simulink model "pilote_hydraulique_Stateflow_0"  (R2020a)
settings: Solver=ode23t  StartTime=0.0  StopTime=1500  RelTol=1e-3  EnableMultiTasking=on
undefined symbols (not defined in the file): sigbuilder_block, X, Y, Z
libraries: sm_lib x295, fl_lib x24, nesl_utility x13, sh_lib x5, simulink x1
(part 1 of 5)
settings Model: Creator=Ivan  LastModifiedBy=ivanl
settings DataIOCC: LimitDataPoints=on  SaveFormat=Array  ReturnWorkspaceOutputs=off
settings OptimizationCC: LifeSpan=inf
settings DebuggingCC: UnderspecifiedInitializationDetection=Classic  MergeDetectMultiDrivingBlocksExec=none  SolverPrmCheckMsg=warning  AllowSymbolicDim=off  StateNameClashWarn=warning  SFUnexpectedBacktrackingDiag=warning  SFNoUnconditionalDefaultTransitionDiag=warning  SFExecutionAtInitializationDiag=none  ArithmeticOperatorsInVariantConditions=warning
settings HardwareCC: ProdBitPerPointer=32  ProdBitPerSizeT=32  ProdBitPerPtrDiffT=32  ProdLargestAtomicFloat=None  ProdIntDivRoundTo=Undefined  ProdEndianess=Unspecified  ProdWordSize=32  ProdHWDeviceType=32-bit Generic
settings ModelReferenceCC: PropagateSignalLabelsOutOfModel=off
settings SFSimCC: SimUseLocalCustomCode=off  CustomCodeUndefinedFunction=UseInterfaceOnly
settings RTWCC: RTWUseLocalCustomCode=off
settings CodeAppCC: StateflowObjectComments=on
settings GRTTargetCC: TargetLangStandard=C89/C90 (ANSI)
settings ConfigComp: CovMetricSettings=dw  CovHtmlReporting=on  CovSaveCumulativeToWorkspaceVar=on  CovSaveSingleToWorkspaceVar=on  CovExternalEMLEnable=off
settings SimscapeCC: SimscapeNormalizeSystem=off  SimscapeLogType=all  SimscapeLogLimitData=off
settings ConfigurationSet: Description=SimMechanics 2G
settings ExplorerConfigSet: InternalSimMechanicsExplorerSettings="<ExplorerConfiguration><canonicalview>default</canonicalview><AnimationSetting><BasePlaybackSpeed>1.0</BasePlaybackSpeed><PlaybackSpeedFactor>16.0</PlaybackSpeedFactor></AnimationSetting><TilePanel><TileInfo><Tiles Columns=\"2\" Count=\"4\" Rows=\"2\"><Column Left=\"2\" Weight=\"0.5\"/><Column Left=\"554\" Weight=\"0.5\"/><Column Left=\"1106\"/><Row Top=\"2\" Weight=\"0.4992\"/><Row Top=\"320\" Weight=\"0.5008\"/><Row Top=\"639\"/><Tile Height=\"1\" Width=\"1\" X=\"0\" Y=\"0\"/><Tile Height=\"1\" Width=\"1\" X=\"0\" Y=\"1\"/><Tile Height=\"1\" Width=\"1\" X=\"1\" Y=\"0\"/><Tile Height=\"1\" Width=\"1\" X=\"1\" Y=\"1\"/></Tiles></TileInfo><SceneInfo><SceneViewer><BGColor><R>0.60000002384185791</R><G>0.60000002384185791</G><B>0.60000002384185791</B></BGColor><Camera><Position><X>-1.4545420789578025</X><Y>-0.47703526853152423</Y><Z>1.053292472596125</Z></Position><Center><X>-1.0755331343287176</X><Y>0.65681441625729753</Y><Z>0.33046154790126991</Z></Center><Up><X>0.31799715127972389</X><Y>0.43179203595848165</Y><Z>0.84405772874893448</Z></Up><Left>-0.52137946486473086</Left><Right>0.52137946486473086</Right><Bottom>-0.12744375988841058</Bottom><Top>0.12744375988841058</Top></Camera></SceneViewer><SceneViewer><BGColor><R>0.60000002384185791</R><G>0.60000002384185791</G><B>0.60000002384185791</B></BGColor><Camera><Position><X>-1.097124655307177</X><Y>0.60879350298107193</Y><Z>1.6773847746848054</Z></Position><Center><X>-1.097124655307177</X><Y>0.60879350298107193</Y><Z>0.3230140209197998</Z></Center><Up><X>0</X><Y>1</Y><Z>-0</Z></Up><Left>-0.52137946486473086</Left><Right>0.52137946486473086</Right><Bottom>-0.19162502065300943</Bottom><Top>0.19162502065300943</Top></Camera></SceneViewer><SceneViewer><BGColor><R>0.60000002384185791</R><G>0.60000002384185791</G><B>0.60000002384185791</B></BGColor><Camera><Position><X>-1.839713975613805</X><Y>1.4497817237667032</Y><Z>1.0667372871108483</Z></Position><Center><X>-1.0007040048852538</X><Y>0.55541256489420043</Y><Z>0.26430212739881542</Z></Center><Up><X>0.29701754457873719</X><Y>-0.46808723288325788</Y><Z>0.83227094183571793</Z></Up><Left>-0.47525307471029621</Left><Right>0.47525307471029621</Right><Bottom>-0.31607583672115108</Bottom><Top>0.31607583672115108</Top></Camera></SceneViewer><SceneViewer><BGColor><R>0.60000002384185791</R><G>0.60000002384185791</G><B>0.60000002384185791</B></BGColor><Camera><Position><X>-0.30663977538297038</X><Y>-0.17371608341982503</Y><Z>1.1012231263046517</Z></Position><Center><X>-1.0848488807678223</X><Y>0.60449302196502686</Y><Z>0.3230140209197998</Z></Center><Up><X>-0.40824829046386307</X><Y>0.40824829046386307</Y><Z>0.81649658092772615</Z></Up><Left>-0.50417031347751617</Left><Right>0.50417031347751617</Right><Bottom>-0.39514026045799255</Bottom><Top>0.39514026045799255</Top></Camera></SceneViewer></SceneInfo></TilePanel></ExplorerConfiguration>"

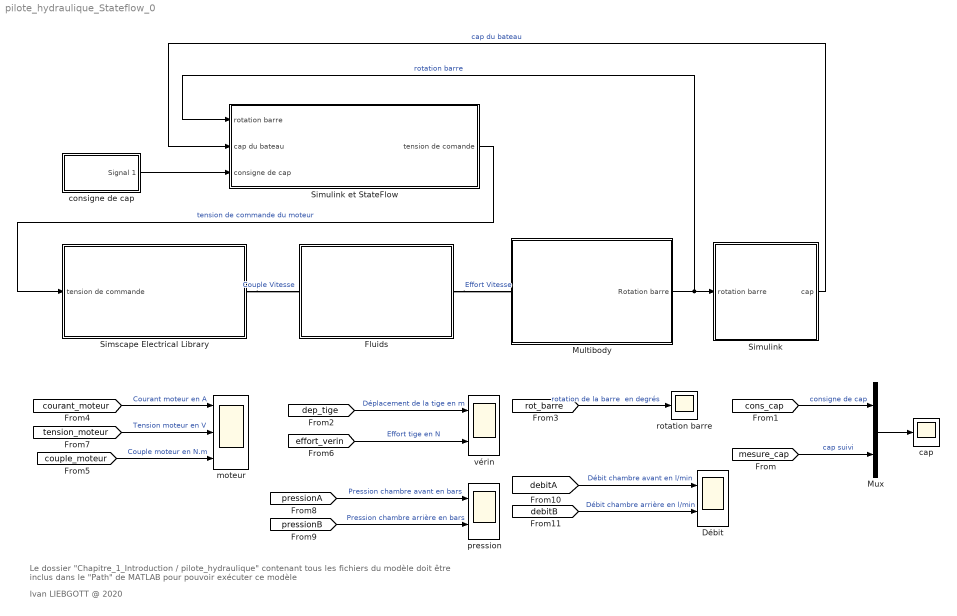
== system pilote_hydraulique_Stateflow_0 ==
  note: Le dossier "Chapitre_1_Introduction / pilote_hydraulique" contenant tous les fichiers du modèle doit être inclus dans le "Path" de MATLAB pour pouvoir exécuter ce modèle
  note: Ivan LIEBGOTT @ 2020
  " moteur" : Scope  NumInputPorts=3
  Débit : Scope  NumInputPorts=2
  Fluids : Subsystem
      mask Display: image('$imagefile'); % Use "Edit Image" on toolstrip to change.
  Multibody : Subsystem
      mask Display: image('$imagefile'); % Use "Edit Image" on toolstrip to change.
  Mux : Mux  Inputs=2
  "Simscape Electrical Library " : Subsystem
      mask Display: image('$imagefile'); % Use "Edit Image" on toolstrip to change.
  Simulink : Subsystem
      mask Display: image('$imagefile'); % Use "Edit Image" on toolstrip to change.
  Simulink et StateFlow : Subsystem
      mask Display: image('$imagefile'); % Use "Edit Image" on toolstrip to change.
  "cap " : Scope
  consigne de cap : Subsystem  Tag=STV Subsys  LoadFcn=sigbuilder_block('load');  StartFcn=sigbuilder_block('start');  StopFcn=sigbuilder_block('stop');  ClipboardFcn=sigbuilder_block('clipboard');  mask(Sigbuilder block){tuvar=[0:10]}
      mask help: Simulink:masks:SigbuilderBlock_MD
      mask init:
      | if ~strcmp(get_param(bdroot(gcbh),'SimulationStatus'),'stopped') tuvar = sigbuilder_block('maskInit'); end
      settings: CopyFcn=sigbuilder_block('copy');  DeleteFcn=sigbuilder_block('delete');  ModelCloseFcn=sigbuilder_block('modelClose');  PreSaveFcn=sigbuilder_block('preSave');  PauseFcn=sigbuilder_block('pause');  ContinueFcn=sigbuilder_block('continue');  NameChangeFcn=sigbuilder_block('namechange');  OpenFcn=sigbuilder_block('open',[-840 183.75 550.5 396 ]);  CloseFcn=sigbuilder_block('close');
      mask Display: plot(0, 0, 100, 100,[2, 2, 32, 32, 2], [68, 8, 8, 68, 68],[32, 2], [38, 38], [32, 19, 2],[53, 60, 44], [32, 17, 17, 2],[16, 16, 31, 31]);txt = getActiveGroup(gcbh);text(2, 100, txt,'verticalAlignment', 'top');
  pression : Scope  NumInputPorts=2
  rotation barre : Scope
  vérin : Scope  NumInputPorts=2
  wires:
  Multibody/1(Rotation barre) -> Simulink/1(rotation barre), Simulink et StateFlow/1(rotation barre)  "rotation barre"
  Mux/1 -> "cap "/1
  [mesure_cap] -> Mux/2  "cap suivi"
  [cons_cap] -> Mux/1  "consigne de cap"
  [dep_tige] -> vérin/1  "Déplacement de la tige en m"
  [rot_barre] -> rotation barre/1  "rotation de la barre  en degrés"
  [courant_moteur] -> " moteur"/1  "Courant moteur en A"
  [couple_moteur] -> " moteur"/3  "Couple moteur en N.m"
  [effort_verin] -> vérin/2  "Effort tige en N"
  consigne de cap/1(Signal 1) -> Simulink et StateFlow/3(consigne de cap)
  Simulink/1(cap) -> Simulink et StateFlow/2(cap du bateau)  "cap du bateau"
  Simulink et StateFlow/1("tension de comande ") -> "Simscape Electrical Library "/1(tension de commande)  "tension de commande du moteur"
  [tension_moteur] -> " moteur"/2  "Tension moteur en V"
  [pressionA] -> pression/1  "Pression chambre avant en bars"
  [pressionB] -> pression/2  "Pression chambre arrière en bars"
  [debitA] -> Débit/1  "Débit chambre avant en l/min"
  [debitB] -> Débit/2  "Débit chambre arrière en l/min"
  connections:
  "Simscape Electrical Library "/RConn1 -- Fluids/LConn1  "Couple Vitesse"
  Fluids/RConn1 -- Multibody/LConn1  "Effort Vitesse"

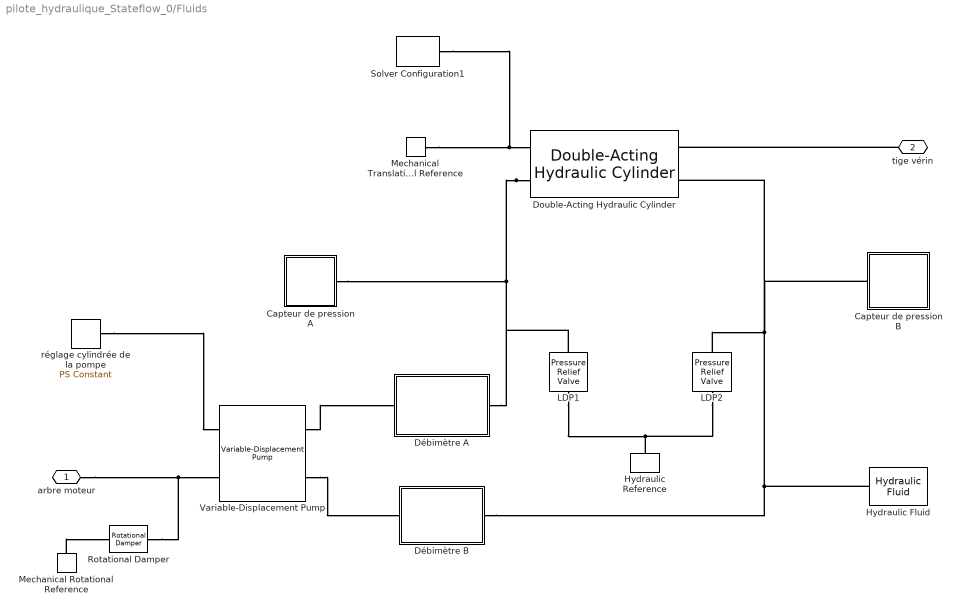
== system pilote_hydraulique_Stateflow_0/Fluids ==
  " LDP1" : sh_lib/Valves/Pressure Control Valves/Pressure Relief Valve  valve_area_spec=1  p_diff_TLU=[30.15e5 : 15e3 : 31.35e5] Pa  area_TLU=[1 : 1 : 9] .* 1e-5 m^2  area_max=1e-4 m^2  pres_set=10e+6 Pa  reg_range=5e+5 Pa  C_d=0.7  A_leak=1e-12 m^2  lam_spec=2  B_lam=0.999  Re_cr=12  dynamic=0  tau=0.1 s  area_init=1e-12 m^2
      settings: SourceProductBaseCode=SH  InternalSimscapePortConfiguration="{\"Bottom\":[],\"Left\":[{\"id\":\"A\",\"label\":\"A\",\"type\":\"foundation.hydraulic.hydraulic\"}],\"Right\":[{\"id\":\"B\",\"label\":\"B\",\"type\":\"foundation.hydraulic.hydraulic\"}],\"Top\":[]}"
  Capteur de pression A : Subsystem
      mask Display: image('$imagefile'); % Use "Edit Image" on toolstrip to change.
  Capteur de pression B : Subsystem
      mask Display: image('$imagefile'); % Use "Edit Image" on toolstrip to change.
  Double-Acting Hydraulic Cylinder : sh_lib/Hydraulic Cylinders/Double-Acting Hydraulic Cylinder  area_A=2e-4 m^2  area_B=2e-4 m^2  stroke=0.3 m  init_pos=0.15 m  dead_vol_A=1e-4 m^3  dead_vol_B=1e-4 m^3  init_pressure_A=0 Pa  init_pressure_B=0 Pa  k_sh=1.4  stiff=1e+6 N/m  D=150 N/(m/s)  hardstop_model=3  transition=0.1 mm  or=1
      settings: SourceProductBaseCode=SH  InternalSimscapePortConfiguration="{\"Bottom\":[],\"Left\":[{\"id\":\"C\",\"label\":\"C\",\"type\":\"foundation.mechanical.translational.translational\"},{\"id\":\"A\",\"label\":\"A\",\"type\":\"foundation.hydraulic.hydraulic\"}],\"Right\":[{\"id\":\"R\",\"label\":\"R\",\"type\":\"foundation.mechanical.translational.translational\"},{\"id\":\"B\",\"label\":\"B\",\"type\":\"foundation.hydraulic.hydraulic\"}],\"Top\":[]}"
  Débimètre A : Subsystem
      mask Display: image('$imagefile'); % Use "Edit Image" on toolstrip to change.
  Débimètre B : Subsystem
      mask Display: image('debimetre.jpg'); % Use "Edit Image" on toolstrip to change.
  Hydraulic Fluid : sh_lib/Hydraulic Utilities/Hydraulic Fluid  DataSource=1  SelFluid=1  SysTemp=60  TrapAir=0.005  ViscDerFactor=1  range_error=2
  Hydraulic Reference : fl_lib/Hydraulic/Hydraulic Elements/Hydraulic Reference
  LDP2 : sh_lib/Valves/Pressure Control Valves/Pressure Relief Valve  valve_area_spec=1  p_diff_TLU=[30.15e5 : 15e3 : 31.35e5] Pa  area_TLU=[1 : 1 : 9] .* 1e-5 m^2  area_max=1e-4 m^2  pres_set=10e+6 Pa  reg_range=5e+5 Pa  C_d=0.7  A_leak=1e-12 m^2  lam_spec=2  B_lam=0.999  Re_cr=12  dynamic=0  tau=0.1 s  area_init=1e-12 m^2
      settings: SourceProductBaseCode=SH  InternalSimscapePortConfiguration="{\"Bottom\":[],\"Left\":[{\"id\":\"A\",\"label\":\"A\",\"type\":\"foundation.hydraulic.hydraulic\"}],\"Right\":[{\"id\":\"B\",\"label\":\"B\",\"type\":\"foundation.hydraulic.hydraulic\"}],\"Top\":[]}"
  Mechanical Rotational Reference : fl_lib/Mechanical/Rotational Elements/Mechanical Rotational Reference
  Mechanical Translational Reference : fl_lib/Mechanical/Translational Elements/Mechanical Translational Reference
  Rotational Damper : fl_lib/Mechanical/Rotational Elements/Rotational Damper  D=0.006 N*m/(rad/s)  w_specify=off  w_priority=None  w=0 rad/s  w_nominal_specify=off  w_nominal_unit=rad/s  w_nominal_value=1  t_specify=off  t_priority=None  t=0 N*m  t_nominal_specify=off  t_nominal_unit=N*m  t_nominal_value=1
  Solver Configuration1 : nesl_utility/Solver Configuration  PhysicalDomain=network_engine_domain  SubClassName=solver  LeftPortType=input  RightPortType=generic  Tones=[]  Harmonics=[]  SimulateNoise=off  Profile=off  UseLocalSampling=off  EnableSwitchedLinearOptims=on  FrequencyDomain=off  UseCCode=off  RelTol=0.001  AbsTol=1e-06  MinStep=1e-09  ToWorkspace=off  RevertToSquareIcSolve=off  NumHomotopyIterations=100  PhasorMode=off  PhasorModeNumHarmonics=1  DoDC=off  ResidualTolerance=1e-09  UseLocalSolver=off  LocalSolverChoice=NE_BACKWARD_EULER_ADVANCER  LocalSolverSampleTime=0.001  DoFixedCost=off  MaxNonlinIter=3  MaxModeIter=2  LinearAlgebra=Sparse  EquationFormulation=NE_TIME_EF  DelaysMemoryBudget=1024  AutomaticFiltering=on  FilteringTimeConstant=0.001  PartitionStorageMethod=AS_NEEDED  PartitionMemoryBudget=1024  PartitionMethod=FAST
  Variable-Displacement Pump : sh_lib/Pumps and Motors/Variable-Displacement Pump  mdl_type=1  stroke_max=1 m  D_max=1.77e-7 m^3/rad  cntrl_mem_tab=[ -0.0075 -0.0025 0 0.0025 0.0075 ] m  displ_tab=[ -5e-6 -3e-6 0 3e-6 5e-6 ] m^3/rad  interp_method=1  extrap_method=1  loss_spec=1  w_nominal=188 rad/s  pr_nominal=1e+8 Pa  visc_nominal=18 cSt  dens_nominal=900 kg/m^3  efficiency_vol=0.85  no_load_torque=0 N*m  torque_pressure_coeff=1*(1.77e-7)*((0.85)/(0.75)-1 ) N*m/Pa  p_diff_eff_TLU=[100000, 1000000, 2000000] Pa  omega_eff_TLU=[25, 50, 100, 200, 300, 400] rad/s  displacement_eff_TLU=[-30, -19, 19, 30] cm^3/rev  vol_eff_TLU=repmat([.816, .908, .954, .977, .981, .984; .325, .663, .831, .916, .925, .946; .137, .568, .78, .892, .893, .91], 1, 1, 4)  mech_eff_TLU=repmat([.996, .996, .996, .996, .996, .996; .988, .989, .989, .989, .989, .99; .981, .981, .982, .982, .983, .984], 1, 1, 4)  p_diff_loss_TLU=[100000, 1000000, 2000000] Pa  omega_loss_TLU=[25, 50, 100, 200, 300, 400] rad/s  displacement_loss_TLU=[-30, -19, 19, 30] cm^3/rev  vol_loss_TLU=repmat([.023, .023, .023, .023, .0285, .032; .0844, .0842, .0845, .084, .1125, .108; .1079, .108, .11, .108, .1605, .18] * 1e-3, 1, 1, 4) m^3/s  mech_loss_TLU=repmat([.002, .002, .002, .002, .002, .002; .0607, .0556, .0556, .0556, .0556, .0505; .1937, .1937, .1833, .1833, .1729, .1626], 1, 1, 4) N*m  pressure_threshold=1e5 Pa  omega_threshold=10 rad/s  displacement_threshold=0.5 cm^3/rev  octant_check=0  pressure_check=0  min_valid_pressure=0 Pa  vol_eff_min=1e-3  vol_eff_max=1  mech_eff_min=1e-3  mech_eff_max=1
      settings: SourceProductBaseCode=SH  InternalSimscapePortConfiguration="{\"Bottom\":[],\"Left\":[{\"id\":\"C\",\"label\":\"C\",\"type\":\"input\"},{\"id\":\"S\",\"label\":\"S\",\"type\":\"foundation.mechanical.rotational.rotational\"}],\"Right\":[{\"id\":\"P\",\"label\":\"P\",\"type\":\"foundation.hydraulic.hydraulic\"},{\"id\":\"T\",\"label\":\"T\",\"type\":\"foundation.hydraulic.hydraulic\"}],\"Top\":[]}"
  réglage cylindrée de la pompe : fl_lib/Physical Signals/Sources/PS Constant  constant=0.4
  arbre moteur : PMIOPort  Side=Left
  tige vérin : PMIOPort  Port=2  Side=Right
  connections:
  arbre moteur/RConn1 -- Rotational Damper/RConn1 -- Variable-Displacement Pump/LConn2
  réglage cylindrée de la pompe/RConn1 -- Variable-Displacement Pump/LConn1
  tige vérin/RConn1 -- Double-Acting Hydraulic Cylinder/RConn1
  Mechanical Translational Reference/LConn1 -- Solver Configuration1/RConn1 -- Double-Acting Hydraulic Cylinder/LConn1
  Hydraulic Fluid/RConn1 -- Débimètre B/RConn1 -- Capteur de pression B/LConn1 -- Double-Acting Hydraulic Cylinder/RConn2 -- LDP2/LConn1
  Hydraulic Reference/LConn1 -- " LDP1"/RConn1 -- LDP2/RConn1
  Mechanical Rotational Reference/LConn1 -- Rotational Damper/LConn1
  Double-Acting Hydraulic Cylinder/LConn2 -- Débimètre A/RConn1 -- " LDP1"/LConn1 -- Capteur de pression A/RConn1
  Variable-Displacement Pump/RConn1 -- Débimètre A/LConn1
  Variable-Displacement Pump/RConn2 -- Débimètre B/LConn1

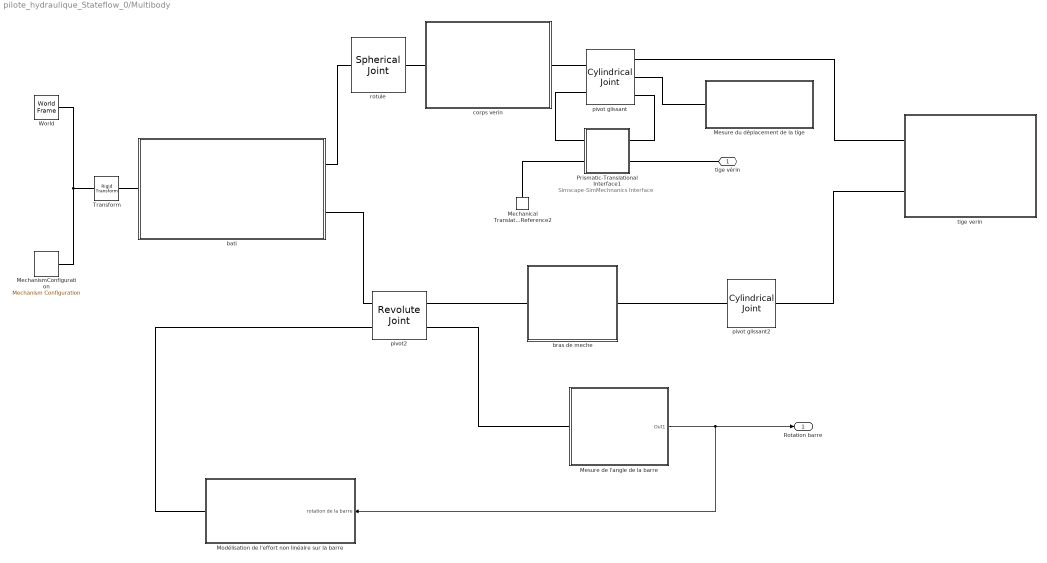
== system pilote_hydraulique_Stateflow_0/Multibody ==
  note: Simscape-SimMechnanics
      |  Interface
  Mechanical Translational Reference2 : fl_lib/Mechanical/Translational Elements/Mechanical Translational Reference
  MechanismConfiguration : sm_lib/Utilities/Mechanism Configuration  UniformGravity=Constant  GravityVector=[0 0 -9.81]  GravityUnits=m/s^2  LinearizationDelta=0.001
  Mesure de l'angle de la barre : Subsystem
      mask Display: image('$imagefile'); % Use "Edit Image" on toolstrip to change.
  Mesure du déplacement de la tige : Subsystem
      mask Display: image('$imagefile'); % Use "Edit Image" on toolstrip to change.
  Modélisation de l'effort non linéaire sur la barre : Subsystem
  Prismatic-Translational Interface1 : Subsystem
  Transform : sm_lib/Frames and Transforms/Rigid Transform  TranslationMethod=Cartesian  TranslationStandardOffset=0  TranslationLengthUnit=mm  TranslationStandardAxis=+Z  TranslationCartesianOffset=[-854.29700000000003 517.99300000000005 336.38900000000001]  TranslationROffset=0  TranslationROffsetUnits=m  TranslationZOffset=0  TranslationZOffsetUnits=m  TranslationThetaOffset=0  TranslationThetaOffsetUnits=deg  RotationMethod=None  RotationAngleUnits=deg  RotationStandardAxis=+Z  RotationAngle=0  RotationArbitraryAxis=[0 0 1]  FollAlignAxisA=+X  BaseAlignAxisA=+Y  FollAlignAxisB=+Y  BaseAlignAxisB=+Z  RotationSequenceAxes=FollowerAxes  RotationSequence=XYX  RotationSequenceAngles=[0 0 0]  RotationSequenceAnglesUnits=deg  RotationMatrix=[1 0 0; 0 1 0; 0 0 1]
  World : sm_lib/Frames and Transforms/World Frame
  bati : Subsystem
      mask Display: image('$imagefile'); % Use "Edit Image" on toolstrip to change.
  bras de meche : Subsystem
      mask Display: image('$imagefile'); % Use "Edit Image" on toolstrip to change.
  corps verin : Subsystem
      mask Display: image('$imagefile'); % Use "Edit Image" on toolstrip to change.
  pivot glissant : sm_lib/Joints/Cylindrical Joint  JointMode=Normal  SenseConstraintForce=off  SenseConstraintForceX=off  SenseConstraintForceY=off  SenseConstraintForceZ=off  SenseConstraintTorque=off  SenseConstraintTorqueX=off  SenseConstraintTorqueY=off  SenseConstraintTorqueZ=off  SenseTotalForce=off  SenseTotalForceX=off  SenseTotalForceY=off  SenseTotalForceZ=off  SenseTotalTorque=off  SenseTotalTorqueX=off  SenseTotalTorqueY=off  SenseTotalTorqueZ=off  CompositeWrenchDir=FollowerOnBase  CompositeWrenchFrame=BaseFrame  PzEquilibriumPosition=0  PzEquilibriumPositionUnits=m  PzSpringStiffness=0  PzSpringStiffnessUnits=N/m  PzDampingCoefficient=0  PzDampingCoefficientUnits=s*N/m  PzTorqueActuationMode=InputTorque  PzMotionActuationMode=ComputedMotion  PzSensePosition=on  PzSenseVelocity=on  PzSenseAcceleration=off  PzSenseTorqueForce=off  PzSenseLowerLimitTorqueForce=off  PzSenseUpperLimitTorqueForce=off  PzLowerLimitSpecify=off  PzLowerLimitBound=-1  PzLowerLimitBoundUnits=m  PzLowerLimitStiffness=1e6  PzLowerLimitStiffnessUnits=N/m  PzLowerLimitDamping=1e3  PzLowerLimitDampingUnits=N/(m/s)  PzLowerLimitTransitionRegionWidth=1e-4  PzLowerLimitTransitionRegionWidthUnits=m  PzUpperLimitSpecify=off  PzUpperLimitBound=1  PzUpperLimitBoundUnits=m  PzUpperLimitStiffness=1e6  PzUpperLimitStiffnessUnits=N/m  PzUpperLimitDamping=1e3  PzUpperLimitDampingUnits=N/(m/s)  PzUpperLimitTransitionRegionWidth=1e-4  PzUpperLimitTransitionRegionWidthUnits=m  PzPositionTargetSpecify=on  PzPositionTargetPriority=Low  PzPositionTargetValue=0  PzPositionTargetValueUnits=m  PzVelocityTargetSpecify=off  PzVelocityTargetPriority=High  PzVelocityTargetValue=0  PzVelocityTargetValueUnits=m/s  RzEquilibriumPosition=0  RzEquilibriumPositionUnits=rad  RzSpringStiffness=0  RzSpringStiffnessUnits=m*N/rad  RzDampingCoefficient=1  RzDampingCoefficientUnits=m*s*N/rad  RzTorqueActuationMode=NoTorque  RzMotionActuationMode=ComputedMotion  RzSensePosition=off  RzSenseVelocity=off  RzSenseAcceleration=off  RzSenseTorqueForce=off  RzSenseLowerLimitTorqueForce=off  RzSenseUpperLimitTorqueForce=off  RzLowerLimitSpecify=off  RzLowerLimitBound=-90  RzLowerLimitBoundUnits=deg  RzLowerLimitStiffness=1e4  RzLowerLimitStiffnessUnits=N*m/deg  RzLowerLimitDamping=10  RzLowerLimitDampingUnits=N*m/(deg/s)  RzLowerLimitTransitionRegionWidth=0.1  RzLowerLimitTransitionRegionWidthUnits=deg  RzUpperLimitSpecify=off  RzUpperLimitBound=90  RzUpperLimitBoundUnits=deg  RzUpperLimitStiffness=1e4  RzUpperLimitStiffnessUnits=N*m/deg  RzUpperLimitDamping=10  RzUpperLimitDampingUnits=N*m/(deg/s)  RzUpperLimitTransitionRegionWidth=0.1  RzUpperLimitTransitionRegionWidthUnits=deg  RzPositionTargetSpecify=on  RzPositionTargetPriority=Low  RzPositionTargetValue=-151.66852375213551  RzPositionTargetValueUnits=deg  RzVelocityTargetSpecify=off  RzVelocityTargetPriority=High  RzVelocityTargetValue=0  RzVelocityTargetValueUnits=deg/s
  pivot glissant2 : sm_lib/Joints/Cylindrical Joint  JointMode=Normal  SenseConstraintForce=off  SenseConstraintForceX=off  SenseConstraintForceY=off  SenseConstraintForceZ=off  SenseConstraintTorque=off  SenseConstraintTorqueX=off  SenseConstraintTorqueY=off  SenseConstraintTorqueZ=off  SenseTotalForce=off  SenseTotalForceX=off  SenseTotalForceY=off  SenseTotalForceZ=off  SenseTotalTorque=off  SenseTotalTorqueX=off  SenseTotalTorqueY=off  SenseTotalTorqueZ=off  CompositeWrenchDir=FollowerOnBase  CompositeWrenchFrame=BaseFrame  PzEquilibriumPosition=0  PzEquilibriumPositionUnits=m  PzSpringStiffness=0  PzSpringStiffnessUnits=N/m  PzDampingCoefficient=0  PzDampingCoefficientUnits=s*N/m  PzTorqueActuationMode=NoTorque  PzMotionActuationMode=ComputedMotion  PzSensePosition=off  PzSenseVelocity=off  PzSenseAcceleration=off  PzSenseTorqueForce=off  PzSenseLowerLimitTorqueForce=off  PzSenseUpperLimitTorqueForce=off  PzLowerLimitSpecify=off  PzLowerLimitBound=-1  PzLowerLimitBoundUnits=m  PzLowerLimitStiffness=1e6  PzLowerLimitStiffnessUnits=N/m  PzLowerLimitDamping=1e3  PzLowerLimitDampingUnits=N/(m/s)  PzLowerLimitTransitionRegionWidth=1e-4  PzLowerLimitTransitionRegionWidthUnits=m  PzUpperLimitSpecify=off  PzUpperLimitBound=1  PzUpperLimitBoundUnits=m  PzUpperLimitStiffness=1e6  PzUpperLimitStiffnessUnits=N/m  PzUpperLimitDamping=1e3  PzUpperLimitDampingUnits=N/(m/s)  PzUpperLimitTransitionRegionWidth=1e-4  PzUpperLimitTransitionRegionWidthUnits=m  PzPositionTargetSpecify=on  PzPositionTargetPriority=Low  PzPositionTargetValue=0  PzPositionTargetValueUnits=m  PzVelocityTargetSpecify=off  PzVelocityTargetPriority=High  PzVelocityTargetValue=0  PzVelocityTargetValueUnits=m/s  RzEquilibriumPosition=0  RzEquilibriumPositionUnits=rad  RzSpringStiffness=0  RzSpringStiffnessUnits=m*N/rad  RzDampingCoefficient=0  RzDampingCoefficientUnits=m*s*N/rad  RzTorqueActuationMode=NoTorque  RzMotionActuationMode=ComputedMotion  RzSensePosition=off  RzSenseVelocity=off  RzSenseAcceleration=off  RzSenseTorqueForce=off  RzSenseLowerLimitTorqueForce=off  RzSenseUpperLimitTorqueForce=off  RzLowerLimitSpecify=off  RzLowerLimitBound=-90  RzLowerLimitBoundUnits=deg  RzLowerLimitStiffness=1e4  RzLowerLimitStiffnessUnits=N*m/deg  RzLowerLimitDamping=10  RzLowerLimitDampingUnits=N*m/(deg/s)  RzLowerLimitTransitionRegionWidth=0.1  RzLowerLimitTransitionRegionWidthUnits=deg  RzUpperLimitSpecify=off  RzUpperLimitBound=90  RzUpperLimitBoundUnits=deg  RzUpperLimitStiffness=1e4  RzUpperLimitStiffnessUnits=N*m/deg  RzUpperLimitDamping=10  RzUpperLimitDampingUnits=N*m/(deg/s)  RzUpperLimitTransitionRegionWidth=0.1  RzUpperLimitTransitionRegionWidthUnits=deg  RzPositionTargetSpecify=on  RzPositionTargetPriority=Low  RzPositionTargetValue=88.917590363493801  RzPositionTargetValueUnits=deg  RzVelocityTargetSpecify=off  RzVelocityTargetPriority=High  RzVelocityTargetValue=0  RzVelocityTargetValueUnits=deg/s
  pivot2 : sm_lib/Joints/Revolute Joint  JointMode=Normal  SenseConstraintForce=off  SenseConstraintForceX=off  SenseConstraintForceY=off  SenseConstraintForceZ=off  SenseConstraintTorque=off  SenseConstraintTorqueX=off  SenseConstraintTorqueY=off  SenseConstraintTorqueZ=off  SenseTotalForce=off  SenseTotalForceX=off  SenseTotalForceY=off  SenseTotalForceZ=off  SenseTotalTorque=off  SenseTotalTorqueX=off  SenseTotalTorqueY=off  SenseTotalTorqueZ=off  CompositeWrenchDir=FollowerOnBase  CompositeWrenchFrame=BaseFrame  EquilibriumPosition=0  EquilibriumPositionUnits=rad  SpringStiffness=0  SpringStiffnessUnits=m*N/rad  DampingCoefficient=0  DampingCoefficientUnits=m*s*N/rad  TorqueActuationMode=InputTorque  MotionActuationMode=ComputedMotion  SensePosition=on  SenseVelocity=off  SenseAcceleration=off  SenseTorqueForce=off  SenseLowerLimitTorqueForce=off  SenseUpperLimitTorqueForce=off  LowerLimitSpecify=off  LowerLimitBound=-90  LowerLimitBoundUnits=deg  LowerLimitStiffness=1e4  LowerLimitStiffnessUnits=N*m/deg  LowerLimitDamping=10  LowerLimitDampingUnits=N*m/(deg/s)  LowerLimitTransitionRegionWidth=0.1  LowerLimitTransitionRegionWidthUnits=deg  UpperLimitSpecify=off  UpperLimitBound=90  UpperLimitBoundUnits=deg  UpperLimitStiffness=1e4  UpperLimitStiffnessUnits=N*m/deg  UpperLimitDamping=10  UpperLimitDampingUnits=N*m/(deg/s)  UpperLimitTransitionRegionWidth=0.1  UpperLimitTransitionRegionWidthUnits=deg  PositionTargetSpecify=on  PositionTargetPriority=Low  PositionTargetValue=91.342079820133691  PositionTargetValueUnits=deg  VelocityTargetSpecify=off  VelocityTargetPriority=High  VelocityTargetValue=0  VelocityTargetValueUnits=deg/s
  rotule : sm_lib/Joints/Spherical Joint  JointMode=Normal  SenseConstraintForce=off  SenseConstraintForceX=off  SenseConstraintForceY=off  SenseConstraintForceZ=off  SenseConstraintTorque=off  SenseConstraintTorqueX=off  SenseConstraintTorqueY=off  SenseConstraintTorqueZ=off  SenseTotalForce=off  SenseTotalForceX=off  SenseTotalForceY=off  SenseTotalForceZ=off  SenseTotalTorque=off  SenseTotalTorqueX=off  SenseTotalTorqueY=off  SenseTotalTorqueZ=off  CompositeWrenchDir=FollowerOnBase  CompositeWrenchFrame=BaseFrame  DefPosRotationMethod=None  DefPosRotationAngleUnits=deg  DefPosRotationStandardAxis=+Z  DefPosRotationAngle=0  DefPosRotationArbitraryAxis=[0 0 1]  DefPosFollAlignAxisA=+X  DefPosBaseAlignAxisA=+Y  DefPosFollAlignAxisB=+Y  DefPosBaseAlignAxisB=+Z  DefPosRotationSequenceAxes=FollowerAxes  DefPosRotationSequence=XYX  DefPosRotationSequenceAngles=[0 0 0]  DefPosRotationSequenceAnglesUnits=deg  DefPosRotationMatrix=[1 0 0; 0 1 0; 0 0 1]  EqPosRotationMethod=None  EqPosRotationAngleUnits=deg  EqPosRotationStandardAxis=+Z  EqPosRotationAngle=0  EqPosRotationArbitraryAxis=[0 0 1]  EqPosFollAlignAxisA=+X  EqPosBaseAlignAxisA=+Y  EqPosFollAlignAxisB=+Y  EqPosBaseAlignAxisB=+Z  EqPosRotationSequenceAxes=FollowerAxes  EqPosRotationSequence=XYX  EqPosRotationSequenceAngles=[0 0 0]  EqPosRotationSequenceAnglesUnits=deg  EqPosRotationMatrix=[1 0 0; 0 1 0; 0 0 1]  SpringStiffness=0  SpringStiffnessUnits=m*N/rad  DampingCoefficient=0  DampingCoefficientUnits=m*s*N/rad  ActuateTorqueX=off  ActuateTorqueY=off  ActuateTorqueZ=off  ActuateTorque=off  TorqueActuationMode=NoTorque  MotionActuationMode=ComputedMotion  ActuationFrame=BaseFrame  SensePosition=off  SenseVelocityX=off  SenseVelocityY=off  SenseVelocityZ=off  SenseVelocity=off  SenseAccelerationX=off  SenseAccelerationY=off  SenseAccelerationZ=off  SenseAcceleration=off  SenseTorqueX=off  SenseTorqueY=off  SenseTorqueZ=off  SenseTorqueForce=off  SenseLowerLimitTorqueMag=off  SenseUpperLimitTorqueMag=off  SensingFrame=FollowerFrame  LowerLimitSpecify=off  LowerLimitBound=15  LowerLimitBoundUnits=deg  LowerLimitStiffness=1e4  LowerLimitStiffnessUnits=N*m/deg  LowerLimitDamping=10  LowerLimitDampingUnits=N*m/(deg/s)  LowerLimitTransitionRegionWidth=0.1  LowerLimitTransitionRegionWidthUnits=deg  UpperLimitSpecify=off  UpperLimitBound=45  UpperLimitBoundUnits=deg  UpperLimitStiffness=1e4  UpperLimitStiffnessUnits=N*m/deg  UpperLimitDamping=10  UpperLimitDampingUnits=N*m/(deg/s)  UpperLimitTransitionRegionWidth=0.1  UpperLimitTransitionRegionWidthUnits=deg  PositionTargetRotationMethod=None  PositionTargetRotationAngleUnits=deg  PositionTargetRotationStandardAxis=+Z  PositionTargetRotationAngle=0  PositionTargetRotationArbitraryAxis=[0 0 1]  PositionTargetFollAlignAxisA=+X  PositionTargetBaseAlignAxisA=+Y  PositionTargetFollAlignAxisB=+Y  PositionTargetBaseAlignAxisB=+Z  PositionTargetRotationSequenceAxes=FollowerAxes  PositionTargetRotationSequence=XYX  PositionTargetRotationSequenceAngles=[0 0 0]  PositionTargetRotationSequenceAnglesUnits=deg  PositionTargetRotationMatrix=[1 0 0; 0 1 0; 0 0 1]  PositionTargetSpecify=off  PositionTargetPriority=High  VelocityTargetValue=[0 0 0]  VelocityTargetValueUnits=deg/s  VelocityTargetSpecify=off  VelocityTargetPriority=High  VelocityTargetInFollowerFrame=on
  tige verin : Subsystem
      mask Display: image('$imagefile'); % Use "Edit Image" on toolstrip to change.
  "tige vérin " : PMIOPort  Side=Left
  Rotation barre : Outport  VectorParamsAs1DForOutWhenUnconnected=off
  wires:
  Mesure de l'angle de la barre/1(Out1) -> Rotation barre/1, Modélisation de l'effort non linéaire sur la barre/1(rotation de la barre)
  connections:
  bati/LConn1 -- Transform/RConn1
  corps verin/LConn1 -- rotule/RConn1
  bati/RConn1 -- rotule/LConn1
  pivot2/RConn1 -- bras de meche/LConn1
  pivot2/LConn1 -- bati/RConn2
  pivot glissant2/LConn1 -- bras de meche/RConn1
  Transform/LConn1 -- World/RConn1 -- MechanismConfiguration/RConn1
  "tige vérin "/RConn1 -- Prismatic-Translational Interface1/LConn2
  Mechanical Translational Reference2/LConn1 -- Prismatic-Translational Interface1/RConn2
  Prismatic-Translational Interface1/RConn1 -- pivot glissant/LConn2
  pivot glissant/RConn3 -- Prismatic-Translational Interface1/LConn1
  pivot glissant2/RConn1 -- tige verin/LConn2
  Modélisation de l'effort non linéaire sur la barre/RConn1 -- pivot2/LConn2
  corps verin/RConn1 -- pivot glissant/LConn1
  pivot glissant/RConn1 -- tige verin/LConn1
  Mesure de l'angle de la barre/LConn1 -- pivot2/RConn2
  Mesure du déplacement de la tige/LConn1 -- pivot glissant/RConn2

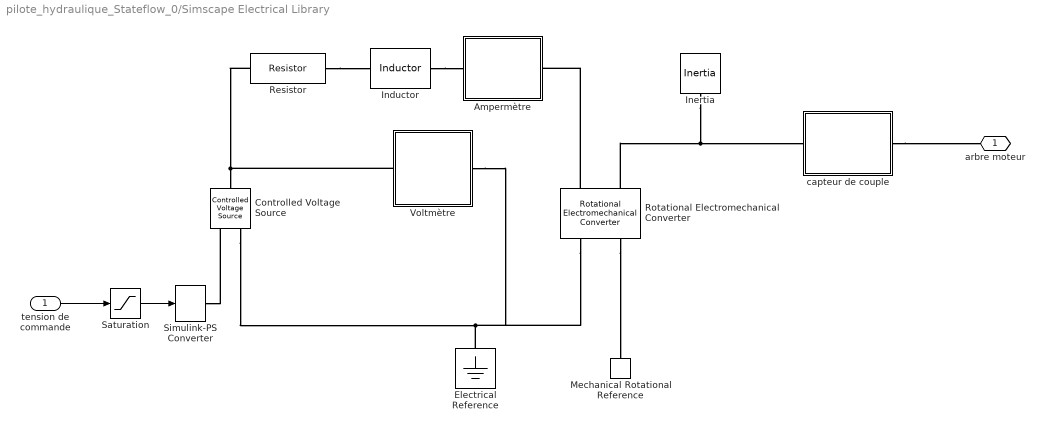
== system pilote_hydraulique_Stateflow_0/Simscape Electrical Library  ==
  tension de commande : Inport
  Ampermètre : Subsystem
      mask Display: image('$imagefile'); % Use "Edit Image" on toolstrip to change.
  Controlled Voltage Source : fl_lib/Electrical/Electrical Sources/Controlled Voltage Source
  Electrical Reference : fl_lib/Electrical/Electrical Elements/Electrical Reference
  Inductor : fl_lib/Electrical/Electrical Elements/Inductor  l=1e-7 H  r=0 Ohm  g=1e-9 1/Ohm  i_specify=off  i_priority=None  i=0 A  i_nominal_specify=off  i_nominal_unit=A  i_nominal_value=1  v_specify=off  v_priority=None  v=0 V  v_nominal_specify=off  v_nominal_unit=V  v_nominal_value=1  i_L_specify=on  i_L_priority=High  i_L=0 A  i_L_nominal_specify=off  i_L_nominal_unit=A  i_L_nominal_value=1
  Inertia : fl_lib/Mechanical/Rotational Elements/Inertia  inertia=0.005 kg*m^2  w_specify=on  w_priority=High  w=0 rad/s  w_nominal_specify=off  w_nominal_unit=rad/s  w_nominal_value=1  t_specify=off  t_priority=None  t=0 N*m  t_nominal_specify=off  t_nominal_unit=N*m  t_nominal_value=1
  Mechanical Rotational Reference : fl_lib/Mechanical/Rotational Elements/Mechanical Rotational Reference
  Resistor : fl_lib/Electrical/Electrical Elements/Resistor  R=0.247 Ohm  i_specify=off  i_priority=None  i=0 A  i_nominal_specify=off  i_nominal_unit=A  i_nominal_value=1  v_specify=off  v_priority=None  v=0 V  v_nominal_specify=off  v_nominal_unit=V  v_nominal_value=1
  Rotational Electromechanical Converter : fl_lib/Electrical/Electrical Elements/Rotational Electromechanical Converter  K=0.047 V/(rad/s)  i_specify=off  i_priority=None  i=0 A  i_nominal_specify=off  i_nominal_unit=A  i_nominal_value=1  v_specify=off  v_priority=None  v=0 V  v_nominal_specify=off  v_nominal_unit=V  v_nominal_value=1  t_specify=off  t_priority=None  t=0 N*m  t_nominal_specify=off  t_nominal_unit=N*m  t_nominal_value=1  w_specify=off  w_priority=None  w=0 rad/s  w_nominal_specify=off  w_nominal_unit=rad/s  w_nominal_value=1
  Saturation : Saturate  UpperLimit=12  LowerLimit=-12
  Simulink-PS Converter : nesl_utility/Simulink-PS Converter  PhysicalDomain=network_engine_domain  SubClassName=ps_input  LeftPortType=input  RightPortType=output  PseudoPeriodic=off  Frequencies=[]  NoiseDistribution=none  NoiseParameters=[]  Unit=V  AffineConversion=off  FilteringAndDerivatives=zero  SimscapeFilterOrder=1  InputFilterTimeConstant=0.001  UdotUserProvided=1
  Voltmètre : Subsystem
      mask Display: image('$imagefile'); % Use "Edit Image" on toolstrip to change.
  capteur de couple : Subsystem
      mask Display: image('$imagefile'); % Use "Edit Image" on toolstrip to change.
  arbre moteur : PMIOPort  Side=Right
  wires:
  tension de commande/1 -> Saturation/1
  Saturation/1 -> Simulink-PS Converter/1
  connections:
  Simulink-PS Converter/RConn1 -- Controlled Voltage Source/RConn1
  Rotational Electromechanical Converter/RConn2 -- Mechanical Rotational Reference/LConn1
  Electrical Reference/LConn1 -- Controlled Voltage Source/RConn2 -- Voltmètre/RConn1 -- Rotational Electromechanical Converter/RConn1
  Resistor/LConn1 -- Voltmètre/LConn1 -- Controlled Voltage Source/LConn1
  Resistor/RConn1 -- Inductor/LConn1
  Inductor/RConn1 -- Ampermètre/LConn1
  Rotational Electromechanical Converter/LConn1 -- Ampermètre/RConn1
  Inertia/LConn1 -- Rotational Electromechanical Converter/LConn2 -- capteur de couple/LConn1
  capteur de couple/RConn1 -- arbre moteur/RConn1

== system pilote_hydraulique_Stateflow_0/Simulink ==
  rotation barre : Inport
  Integrator : Integrator
  Perturbation : Subsystem
      mask Display: image('$imagefile'); % Use "Edit Image" on toolstrip to change.
  Sum : Sum  Inputs=-+|
  Transfer Fcn1 : TransferFcn  Numerator=[0.005]  Denominator=[1 0.1]
  cap : Outport  VectorParamsAs1DForOutWhenUnconnected=off
  wires:
  rotation barre/1 -> Transfer Fcn1/1
  Integrator/1 -> cap/1
  Sum/1 -> Integrator/1
  Transfer Fcn1/1 -> Sum/2
  Perturbation/1(Out1) -> Sum/1

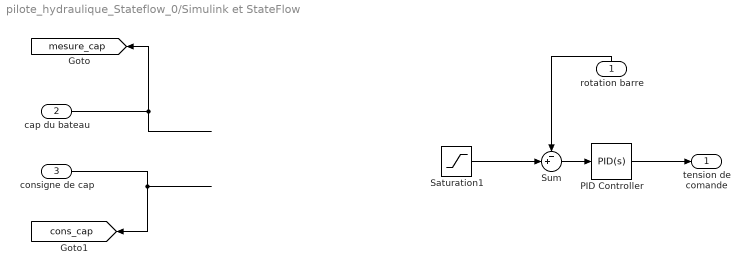
== system pilote_hydraulique_Stateflow_0/Simulink et StateFlow ==
  rotation barre : Inport
  cap du bateau : Inport  Port=2
  consigne de cap : Inport  Port=3
  PID Controller : simulink/Continuous/PID Controller  Controller=PID  Form=Parallel  TimeDomain=Continuous-time  UseExternalTs=off  SampleTime=-1  IntegratorMethod=Forward Euler  FilterMethod=Forward Euler  ControllerParametersSource=internal  P=0.5  I=0.001  D=0  UseFilter=on  N=100  TunerSelectOption=Transfer Function Based (PID Tuner App)  InitialConditionSource=internal  InitialConditionForIntegrator=0  InitialConditionForFilter=0  DifferentiatorICPrevScaledInput=0  ExternalReset=none  TrackingMode=off  Kt=1  LimitOutput=off  UpperSaturationLimit=inf  LowerSaturationLimit=-inf  LinearizeAsGain=on  AntiWindupMode=none  Kb=1  POutMin=[]  POutMax=[]  IOutMin=[]  IOutMax=[]  DOutMin=[]  DOutMax=[]  NOutMin=[]  NOutMax=[]  SumOutMin=[]  SumOutMax=[]  SaturationOutMin=[]  SaturationOutMax=[]  PParamMin=[]  PParamMax=[]  IParamMin=[]  IParamMax=[]  DParamMin=[]  DParamMax=[]  NParamMin=[]  NParamMax=[]  KbParamMin=[]  KbParamMax=[]  KtParamMin=[]  KtParamMax=[]  KbOutMin=[]  KbOutMax=[]  KtOutMin=[]  KtOutMax=[]  IntegratorOutMin=[]  IntegratorOutMax=[]  FilterOutMin=[]  FilterOutMax=[]  SumI1OutMin=[]  SumI1OutMax=[]  SumI2OutMin=[]  SumI2OutMax=[]  SumI3OutMin=[]  SumI3OutMax=[]  SumI4OutMin=[]  SumI4OutMax=[]  SumDOutMin=[]  SumDOutMax=[]  DifferentiatorOutMin=[]  DifferentiatorOutMax=[]  FilterDiffOutCoefMin=[]  FilterDiffOutCoefMax=[]  ReciprocalOutMin=[]  ReciprocalOutMax=[]  SumDenOutMin=[]  SumDenOutMax=[]  SumNumOutMin=[]  SumNumOutMax=[]  DivideOutMin=[]  DivideOutMax=[]  UdiffTsProdOutMin=[]  UdiffTsProdOutMax=[]  NTsProdOutMin=[]  NTsProdOutMax=[]  UintegralTsProdOutMin=[]  UintegralTsProdOutMax=[]  UngainTsProdOutMin=[]  UngainTsProdOutMax=[]  IntegratorContinuousStateAttributes=''  IntegratorStateMustResolveToSignalObject=off  IntegratorRTWStateStorageClass=Auto  FilterContinuousStateAttributes=''  FilterStateMustResolveToSignalObject=off  FilterRTWStateStorageClass=Auto  ParallelPVariant=InternalParameters  IdealPVariant=Disabled  IVariant=InternalParameters  DVariant=InternalParameters  IntegratorVariant=Continuous  SatVariant=Disabled  AWVariant=Passthrough  PCopyVariant=Disabled  TRVariant=Disabled  FdbkBlocksVariant=Forward  IdealPFdbkVariant=Disabled  SatFdbkVariant=Disabled  DerivativeFilterVariant=ContFilter  NVariant=InternalParameters  NCopyVariant=Disabled  FilterICVariant=InternalICsFilter  IntegratorICVariant=InternalICs  ExternalResetVariant=Disabled  TRSumVariant=Passthrough  SumFdbkVariant=Disabled  SumVariant=Sum_PID  TsampFilterVariant=InternalTs  TsampNgainVariant=Passthrough  TsampIntegralVariant=Passthrough
  Saturation1 : Saturate  UpperLimit=25  LowerLimit=-25
  Sum : Sum  Inputs=-+|
  "tension de comande " : Outport  VectorParamsAs1DForOutWhenUnconnected=off
  tag scope: cons_cap=global, mesure_cap=global
  wires:
  rotation barre/1 -> Sum/1
  consigne de cap/1 -> [cons_cap]
  cap du bateau/1 -> [mesure_cap]
  Sum/1 -> PID Controller/1
  PID Controller/1 -> "tension de comande "/1
  ? -> Saturation1/1
  Saturation1/1 -> Sum/2

== system pilote_hydraulique_Stateflow_0/consigne de cap ==
  Demux : Demux  Tag=STV Demux  Outputs=1
      settings: DisplayOption=none
  FromWs : FromWorkspace  Tag=STV FromWs  VariableName=tuvar
      SigBuilderData=|
      | common.afterFinalStr = 'Extrapolate'
      | common.sampleTime = 0
      | dataSet.timeRange = [0 1500]
      | dataSet.name = 'Group 1'
      | sbobj.Groups.Name = 'Group 1'
      | sbobj.Groups.Signals.Name = 'Signal 1'
      | sbobj.Groups.Signals.XData = [0 502 502 1500]
      | sbobj.Groups.Signals.YData = [20 20 -40 -40]
      | sbobj.Groups.TimeRange = [0 1500]
  Signal 1 : Outport  Tag=STV Outport  VectorParamsAs1DForOutWhenUnconnected=off
  wires:
  Demux/1 -> Signal 1/1
  FromWs/1 -> Demux/1

== system pilote_hydraulique_Stateflow_0/Fluids/Capteur de pression A ==
  Hydraulic Pressure Sensor : fl_lib/Hydraulic/Hydraulic Sensors/Hydraulic Pressure Sensor
  Hydraulic Reference1 : fl_lib/Hydraulic/Hydraulic Elements/Hydraulic Reference
  PS-Simulink Converter2 : nesl_utility/PS-Simulink Converter  PhysicalDomain=network_engine_domain  SubClassName=ps_output  LeftPortType=input  RightPortType=output  PseudoPeriodic=off  Frequencies=[]  Unit=bar  AffineConversion=off
  Conn1 : PMIOPort  Side=Right
  tag scope: pressionA=global
  wires:
  PS-Simulink Converter2/1 -> [pressionA]
  connections:
  Hydraulic Pressure Sensor/LConn1 -- Conn1/RConn1
  PS-Simulink Converter2/LConn1 -- Hydraulic Pressure Sensor/RConn2
  Hydraulic Reference1/LConn1 -- Hydraulic Pressure Sensor/RConn1

== system pilote_hydraulique_Stateflow_0/Fluids/Capteur de pression B ==
  Hydraulic Pressure Sensor1 : fl_lib/Hydraulic/Hydraulic Sensors/Hydraulic Pressure Sensor
  Hydraulic Reference2 : fl_lib/Hydraulic/Hydraulic Elements/Hydraulic Reference
  PS-Simulink Converter3 : nesl_utility/PS-Simulink Converter  PhysicalDomain=network_engine_domain  SubClassName=ps_output  LeftPortType=input  RightPortType=output  PseudoPeriodic=off  Frequencies=[]  Unit=bar  AffineConversion=off
  Conn1 : PMIOPort  Side=Left
  tag scope: pressionB=global
  wires:
  PS-Simulink Converter3/1 -> [pressionB]
  connections:
  Hydraulic Reference2/LConn1 -- Hydraulic Pressure Sensor1/RConn1
  Hydraulic Pressure Sensor1/RConn2 -- PS-Simulink Converter3/LConn1
  Hydraulic Pressure Sensor1/LConn1 -- Conn1/RConn1

== system pilote_hydraulique_Stateflow_0/Fluids/Débimètre A ==
  Hydraulic Flow Rate Sensor : fl_lib/Hydraulic/Hydraulic Sensors/Hydraulic Flow Rate Sensor
  PS-Simulink Converter4 : nesl_utility/PS-Simulink Converter  PhysicalDomain=network_engine_domain  SubClassName=ps_output  LeftPortType=input  RightPortType=output  PseudoPeriodic=off  Frequencies=[]  Unit=l/min  AffineConversion=off
  Conn1 : PMIOPort  Side=Right
  Conn2 : PMIOPort  Port=2  Side=Left
  tag scope: debitA=global
  wires:
  PS-Simulink Converter4/1 -> [debitA]
  connections:
  Conn2/RConn1 -- Hydraulic Flow Rate Sensor/LConn1
  Hydraulic Flow Rate Sensor/RConn1 -- PS-Simulink Converter4/LConn1
  Hydraulic Flow Rate Sensor/RConn2 -- Conn1/RConn1

== system pilote_hydraulique_Stateflow_0/Fluids/Débimètre B ==
  Hydraulic Flow Rate Sensor1 : fl_lib/Hydraulic/Hydraulic Sensors/Hydraulic Flow Rate Sensor
  PS-Simulink Converter5 : nesl_utility/PS-Simulink Converter  PhysicalDomain=network_engine_domain  SubClassName=ps_output  LeftPortType=input  RightPortType=output  PseudoPeriodic=off  Frequencies=[]  Unit=l/min  AffineConversion=off
  Conn1 : PMIOPort  Side=Right
  Conn2 : PMIOPort  Port=2  Side=Left
  tag scope: debitB=global
  wires:
  PS-Simulink Converter5/1 -> [debitB]
  connections:
  Conn2/RConn1 -- Hydraulic Flow Rate Sensor1/LConn1
  Hydraulic Flow Rate Sensor1/RConn1 -- PS-Simulink Converter5/LConn1
  Hydraulic Flow Rate Sensor1/RConn2 -- Conn1/RConn1

== system pilote_hydraulique_Stateflow_0/Multibody/Mesure de l'angle de la barre ==
  PS-Simulink Converter : nesl_utility/PS-Simulink Converter  PhysicalDomain=network_engine_domain  SubClassName=ps_output  LeftPortType=input  RightPortType=output  PseudoPeriodic=off  Frequencies=[]  Unit=deg  AffineConversion=off
  Sum : Sum  Inputs=|+-
  offset barre : Constant  Value=91.342079820133691
  Conn1 : PMIOPort  Side=Left
  Out1 : Outport  VectorParamsAs1DForOutWhenUnconnected=off
  tag scope: rot_barre=global
  wires:
  PS-Simulink Converter/1 -> Sum/1
  offset barre/1 -> Sum/2
  Sum/1 -> [rot_barre], Out1/1
  connections:
  PS-Simulink Converter/LConn1 -- Conn1/RConn1

== system pilote_hydraulique_Stateflow_0/Multibody/Mesure du déplacement de la tige ==
  PS-Simulink Converter1 : nesl_utility/PS-Simulink Converter  PhysicalDomain=network_engine_domain  SubClassName=ps_output  LeftPortType=input  RightPortType=output  PseudoPeriodic=off  Frequencies=[]  Unit=m  AffineConversion=off
  Conn1 : PMIOPort  Side=Left
  tag scope: dep_tige=global
  wires:
  PS-Simulink Converter1/1 -> [dep_tige]
  connections:
  PS-Simulink Converter1/LConn1 -- Conn1/RConn1

== system pilote_hydraulique_Stateflow_0/Multibody/Modélisation de l'effort non linéaire sur la barre ==
  rotation de la barre : Inport
  1-D Lookup Table1 : Lookup_n-D  NumberOfTableDimensions=1  BreakpointsForDimension1=[0 5 10 15 20 25 30]  Table=[0 2.5 5 10 30 60 100]  RndMeth=Simplest  InputSameDT=on
  Gain3 : Gain  Gain=-20
  Scope : Scope
  Simulink-PS Converter : nesl_utility/Simulink-PS Converter  PhysicalDomain=network_engine_domain  SubClassName=ps_input  LeftPortType=input  RightPortType=output  PseudoPeriodic=off  Frequencies=[]  NoiseDistribution=none  NoiseParameters=[]  Unit=1  AffineConversion=off  FilteringAndDerivatives=zero  SimscapeFilterOrder=1  InputFilterTimeConstant=0.001  UdotUserProvided=1
  Couple resistant : PMIOPort  Side=Right
  wires:
  1-D Lookup Table1/1 -> Gain3/1
  rotation de la barre/1 -> 1-D Lookup Table1/1
  Gain3/1 -> Simulink-PS Converter/1, Scope/1
  connections:
  Simulink-PS Converter/RConn1 -- Couple resistant/RConn1

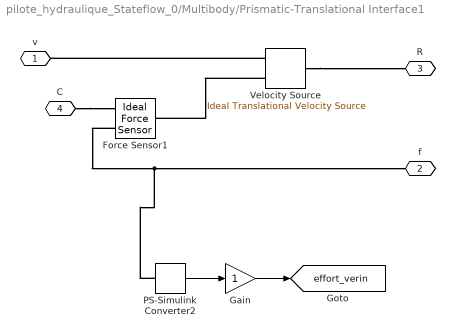
== system pilote_hydraulique_Stateflow_0/Multibody/Prismatic-Translational Interface1 ==
  Force Sensor1 : fl_lib/Mechanical/Mechanical Sensors/Ideal Force Sensor
  Gain : Gain
  PS-Simulink Converter2 : nesl_utility/PS-Simulink Converter  PhysicalDomain=network_engine_domain  SubClassName=ps_output  LeftPortType=input  RightPortType=output  PseudoPeriodic=off  Frequencies=[]  Unit=N  AffineConversion=off
  Velocity Source : fl_lib/Mechanical/Mechanical Sources/Ideal Translational Velocity Source
  v : PMIOPort  Side=Left
  f : PMIOPort  Port=2  Side=Right
  R : PMIOPort  Port=3  Side=Left
  C : PMIOPort  Port=4  Side=Right
  tag scope: effort_verin=global
  wires:
  PS-Simulink Converter2/1 -> Gain/1
  Gain/1 -> [effort_verin]
  connections:
  Velocity Source/LConn1 -- R/RConn1
  Velocity Source/RConn1 -- v/RConn1
  Force Sensor1/RConn2 -- PS-Simulink Converter2/LConn1 -- f/RConn1
  C/RConn1 -- Force Sensor1/RConn1
  Velocity Source/RConn2 -- Force Sensor1/LConn1

== system pilote_hydraulique_Stateflow_0/Multibody/bati ==
  AP_Cadre_2_RIGID : Subsystem
  AP_Platine_2_RIGID : Subsystem
  ReferenceFrame : sm_lib/Frames and Transforms/Reference Frame
  Transform : sm_lib/Frames and Transforms/Rigid Transform  TranslationMethod=Cartesian  TranslationStandardOffset=0  TranslationLengthUnit=mm  TranslationStandardAxis=+Z  TranslationCartesianOffset=[0 -3.5527136788005009e-15 26.61639999999997]  TranslationROffset=0  TranslationROffsetUnits=m  TranslationZOffset=0  TranslationZOffsetUnits=m  TranslationThetaOffset=0  TranslationThetaOffsetUnits=deg  RotationMethod=ArbitraryAxis  RotationAngleUnits=rad  RotationStandardAxis=+Z  RotationAngle=5.5511151231257827e-17  RotationArbitraryAxis=[-0 -1 0]  FollAlignAxisA=+X  BaseAlignAxisA=+Y  FollAlignAxisB=+Y  BaseAlignAxisB=+Z  RotationSequenceAxes=FollowerAxes  RotationSequence=XYX  RotationSequenceAngles=[0 0 0]  RotationSequenceAnglesUnits=deg  RotationMatrix=[1 0 0; 0 1 0; 0 0 1]
  Transform1 : sm_lib/Frames and Transforms/Rigid Transform  TranslationMethod=Cartesian  TranslationStandardOffset=0  TranslationLengthUnit=mm  TranslationStandardAxis=+Z  TranslationCartesianOffset=[-593.50000000000011 155 69]  TranslationROffset=0  TranslationROffsetUnits=m  TranslationZOffset=0  TranslationZOffsetUnits=m  TranslationThetaOffset=0  TranslationThetaOffsetUnits=deg  RotationMethod=ArbitraryAxis  RotationAngleUnits=rad  RotationStandardAxis=+Z  RotationAngle=0  RotationArbitraryAxis=[0 0 0]  FollAlignAxisA=+X  BaseAlignAxisA=+Y  FollAlignAxisB=+Y  BaseAlignAxisB=+Z  RotationSequenceAxes=FollowerAxes  RotationSequence=XYX  RotationSequenceAngles=[0 0 0]  RotationSequenceAnglesUnits=deg  RotationMatrix=[1 0 0; 0 1 0; 0 0 1]
  F2 : PMIOPort  Side=Left
  F1 : PMIOPort  Port=2  Side=Right
  F : PMIOPort  Port=3  Side=Right
  connections:
  AP_Platine_2_RIGID/RConn1 -- AP_Cadre_2_RIGID/RConn1 -- Transform/LConn1 -- Transform1/LConn1 -- F2/RConn1 -- ReferenceFrame/RConn1
  Transform/RConn1 -- F/RConn1
  Transform1/RConn1 -- F1/RConn1

== system pilote_hydraulique_Stateflow_0/Multibody/bras de meche ==
  AP_BrasMeche_1_RIGID : Subsystem
  ArbreMeche_1_RIGID : Subsystem
  ReferenceFrame : sm_lib/Frames and Transforms/Reference Frame
  Transform : sm_lib/Frames and Transforms/Rigid Transform  TranslationMethod=Cartesian  TranslationStandardOffset=0  TranslationLengthUnit=mm  TranslationStandardAxis=+Z  TranslationCartesianOffset=[180 0 27]  TranslationROffset=0  TranslationROffsetUnits=m  TranslationZOffset=0  TranslationZOffsetUnits=m  TranslationThetaOffset=0  TranslationThetaOffsetUnits=deg  RotationMethod=ArbitraryAxis  RotationAngleUnits=rad  RotationStandardAxis=+Z  RotationAngle=3.1415926535897931  RotationArbitraryAxis=[1 0 0]  FollAlignAxisA=+X  BaseAlignAxisA=+Y  FollAlignAxisB=+Y  BaseAlignAxisB=+Z  RotationSequenceAxes=FollowerAxes  RotationSequence=XYX  RotationSequenceAngles=[0 0 0]  RotationSequenceAnglesUnits=deg  RotationMatrix=[1 0 0; 0 1 0; 0 0 1]
  Transform1 : sm_lib/Frames and Transforms/Rigid Transform  TranslationMethod=Cartesian  TranslationStandardOffset=0  TranslationLengthUnit=mm  TranslationStandardAxis=+Z  TranslationCartesianOffset=[0 0 -30.883600000000001]  TranslationROffset=0  TranslationROffsetUnits=m  TranslationZOffset=0  TranslationZOffsetUnits=m  TranslationThetaOffset=0  TranslationThetaOffsetUnits=deg  RotationMethod=ArbitraryAxis  RotationAngleUnits=rad  RotationStandardAxis=+Z  RotationAngle=5.5511151231257821e-17  RotationArbitraryAxis=[-0.99972567740849283 0.02342156976230159 -6.4990081917701904e-19]  FollAlignAxisA=+X  BaseAlignAxisA=+Y  FollAlignAxisB=+Y  BaseAlignAxisB=+Z  RotationSequenceAxes=FollowerAxes  RotationSequence=XYX  RotationSequenceAngles=[0 0 0]  RotationSequenceAnglesUnits=deg  RotationMatrix=[1 0 0; 0 1 0; 0 0 1]
  Transform2 : sm_lib/Frames and Transforms/Rigid Transform  TranslationMethod=Cartesian  TranslationStandardOffset=0  TranslationLengthUnit=mm  TranslationStandardAxis=+Z  TranslationCartesianOffset=[0 0 -168]  TranslationROffset=0  TranslationROffsetUnits=m  TranslationZOffset=0  TranslationZOffsetUnits=m  TranslationThetaOffset=0  TranslationThetaOffsetUnits=deg  RotationMethod=None  RotationAngleUnits=deg  RotationStandardAxis=+Z  RotationAngle=0  RotationArbitraryAxis=[0 0 1]  FollAlignAxisA=+X  BaseAlignAxisA=+Y  FollAlignAxisB=+Y  BaseAlignAxisB=+Z  RotationSequenceAxes=FollowerAxes  RotationSequence=XYX  RotationSequenceAngles=[0 0 0]  RotationSequenceAnglesUnits=deg  RotationMatrix=[1 0 0; 0 1 0; 0 0 1]
  F1 : PMIOPort  Side=Left
  F : PMIOPort  Port=2  Side=Right
  connections:
  ReferenceFrame/RConn1 -- AP_BrasMeche_1_RIGID/RConn1 -- Transform1/LConn1 -- Transform2/LConn1 -- Transform/LConn1
  Transform/RConn1 -- F/RConn1
  Transform1/RConn1 -- F1/RConn1
  ArbreMeche_1_RIGID/LConn1 -- Transform2/RConn1
